simulink model "HW3-5"  (R2024b)
settings: Solver=FixedStepDiscrete  StartTime=0.0  StopTime=10  FixedStep=dt  RelTol=1e-3
PreLoadFcn:
  | run('params.m');
undefined symbols (not defined in the file or in its folder): DiscIntNeverNeededParam, dspblkCoreblockFVToolHelper, dt, gcbh, K1, K2, K3, r, R, tau1, tau2, tau3, th0, vx_d, vy_d, w_d, x0, y0
libraries: simulink x3, slpidlib x3
settings Model: Creator=obhav  LastModifiedBy=obhav
settings DataIOCC: ReturnWorkspaceOutputs=off

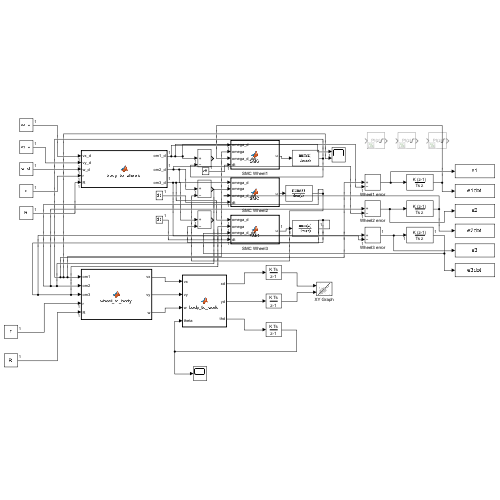
[thumbnail: Simulink's stored preview of the top-level diagram]
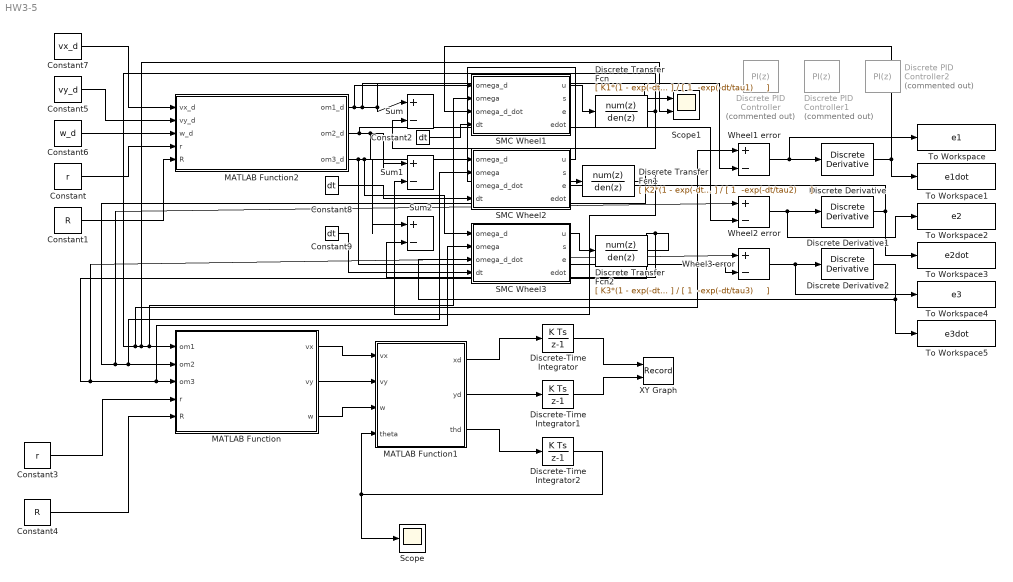
== system HW3-5 ==
  Constant : Constant  Value=r
  Constant1 : Constant  Value=R
  Constant2 : Constant  Value=dt
  Constant3 : Constant  Value=r
  Constant4 : Constant  Value=R
  Constant5 : Constant  Value=vy_d
  Constant6 : Constant  Value=w_d
  Constant7 : Constant  Value=vx_d
  Constant8 : Constant  Value=dt
  Constant9 : Constant  Value=dt
  Discrete Transfer Fcn : DiscreteTransferFcn  LoadFcn=dspblkCoreblockFVToolHelper(gcbh,'load');  Numerator=[ K1*(1 - exp(-dt/tau1)) ]  Denominator="[ 1  -exp(-dt/tau1)     ]"
      settings: CopyFcn=dspblkCoreblockFVToolHelper(gcbh,'copy');  DeleteFcn=dspblkCoreblockFVToolHelper(gcbh,'close');  ModelCloseFcn=dspblkCoreblockFVToolHelper(gcbh,'close');  PreSaveFcn=dspblkCoreblockFVToolHelper(gcbh,'presave');  PostSaveFcn=dspblkCoreblockFVToolHelper(gcbh,'postsave');  CloseFcn=dspblkCoreblockFVToolHelper(gcbh,'close');
  Discrete Transfer Fcn1 : DiscreteTransferFcn  LoadFcn=dspblkCoreblockFVToolHelper(gcbh,'load');  Numerator=[ K2*(1 - exp(-dt/tau2)) ]  Denominator="[ 1  -exp(-dt/tau2)     ]"
      settings: CopyFcn=dspblkCoreblockFVToolHelper(gcbh,'copy');  DeleteFcn=dspblkCoreblockFVToolHelper(gcbh,'close');  ModelCloseFcn=dspblkCoreblockFVToolHelper(gcbh,'close');  PreSaveFcn=dspblkCoreblockFVToolHelper(gcbh,'presave');  PostSaveFcn=dspblkCoreblockFVToolHelper(gcbh,'postsave');  CloseFcn=dspblkCoreblockFVToolHelper(gcbh,'close');
  Discrete Transfer Fcn2 : DiscreteTransferFcn  LoadFcn=dspblkCoreblockFVToolHelper(gcbh,'load');  Numerator=[ K3*(1 - exp(-dt/tau3)) ]  Denominator="[ 1  -exp(-dt/tau3)     ]"
      settings: CopyFcn=dspblkCoreblockFVToolHelper(gcbh,'copy');  DeleteFcn=dspblkCoreblockFVToolHelper(gcbh,'close');  ModelCloseFcn=dspblkCoreblockFVToolHelper(gcbh,'close');  PreSaveFcn=dspblkCoreblockFVToolHelper(gcbh,'presave');  PostSaveFcn=dspblkCoreblockFVToolHelper(gcbh,'postsave');  CloseFcn=dspblkCoreblockFVToolHelper(gcbh,'close');
  Discrete Derivative : simulink/Discrete/Discrete Derivative  gainval=1.0  ICPrevScaledInput=0.0  OutMin=[]  OutMax=[]  OutDataType=fixdt(1, 16)  OutScaling=2^-10  DoSatur=off
  Discrete Derivative1 : simulink/Discrete/Discrete Derivative  gainval=1.0  ICPrevScaledInput=0.0  OutMin=[]  OutMax=[]  OutDataType=fixdt(1, 16)  OutScaling=2^-10  DoSatur=off
  Discrete Derivative2 : simulink/Discrete/Discrete Derivative  gainval=1.0  ICPrevScaledInput=0.0  OutMin=[]  OutMax=[]  OutDataType=fixdt(1, 16)  OutScaling=2^-10  DoSatur=off
  Discrete PID Controller : slpidlib/PID Controller  Commented=on  Controller=PI  Form=Parallel  TimeDomain=Discrete-time  UseExternalTs=off  SampleTime=dt  IntegratorMethod=Forward Euler  FilterMethod=Forward Euler  ControllerParametersSource=internal  P=5  I=50  UseKiTs=off  D=0  UseExternalDerivativeSource=off  N=100  UseFilter=on  TunerSelectOption=Transfer Function Based (PID Tuner App)  InitialConditionSource=internal  InitialConditionForIntegrator=0  InitialConditionForFilter=0  DifferentiatorICPrevScaledInput=0  ExternalReset=none  TrackingMode=off  Kt=1  LimitOutput=on  SatLimitsSource=internal  UpperSaturationLimit=10  LowerSaturationLimit=-10  LinearizeAsGain=off  AntiWindupMode=clamping  Kb=1  LimitIntegrator=off  UpperIntegratorSaturationLimit=inf  LowerIntegratorSaturationLimit=-inf  POutMin=[]  POutMax=[]  IOutMin=[]  IOutMax=[]  DOutMin=[]  DOutMax=[]  NOutMin=[]  NOutMax=[]  SumOutMin=[]  SumOutMax=[]  SaturationOutMin=[]  SaturationOutMax=[]  PParamMin=[]  PParamMax=[]  IParamMin=[]  IParamMax=[]  DParamMin=[]  DParamMax=[]  NParamMin=[]  NParamMax=[]  KbParamMin=[]  KbParamMax=[]  KtParamMin=[]  KtParamMax=[]  KbOutMin=[]  KbOutMax=[]  KtOutMin=[]  KtOutMax=[]  IntegratorOutMin=[]  IntegratorOutMax=[]  FilterOutMin=[]  FilterOutMax=[]  SumI1OutMin=[]  SumI1OutMax=[]  SumI2OutMin=[]  SumI2OutMax=[]  SumI3OutMin=[]  SumI3OutMax=[]  SumI4OutMin=[]  SumI4OutMax=[]  SumDOutMin=[]  SumDOutMax=[]  DifferentiatorOutMin=[]  DifferentiatorOutMax=[]  FilterDiffOutCoefMin=[]  FilterDiffOutCoefMax=[]  ReciprocalOutMin=[]  ReciprocalOutMax=[]  SumDenOutMin=[]  SumDenOutMax=[]  SumNumOutMin=[]  SumNumOutMax=[]  DivideOutMin=[]  DivideOutMax=[]  UdiffTsProdOutMin=[]  UdiffTsProdOutMax=[]  NTsProdOutMin=[]  NTsProdOutMax=[]  UintegralTsProdOutMin=[]  UintegralTsProdOutMax=[]  UngainTsProdOutMin=[]  UngainTsProdOutMax=[]  ClampingZeroOutDataTypeStr=Inherit: Inherit via back propagation  ClampingZeroOutMin=[]  ClampingZeroOutMax=[]  FilterDenConstantOutDataTypeStr=Inherit: Inherit via back propagation  FilterDenConstantOutMin=[]  FilterDenConstantOutMax=[]  PCopyOutDataTypeStr=Inherit: Inherit via back propagation  PCopyOutMin=[]  PCopyOutMax=[]  NCopyOutDataTypeStr=Inherit: Inherit via back propagation  NCopyOutMin=[]  NCopyOutMax=[]  IntegratorContinuousStateAttributes=''  IntegratorStateMustResolveToSignalObject=off  IntegratorRTWStateStorageClass=Auto  FilterContinuousStateAttributes=''  FilterStateMustResolveToSignalObject=off  FilterRTWStateStorageClass=Auto  ParallelPVariant=InternalParameters  IdealPVariant=Disabled  IVariant=InternalParameters  DVariant=Disabled  IntegratorVariant=Discrete  SatVariant=Enabled  AWVariant=DiscClampingParallel  PCopyVariant=Disabled  TRVariant=Disabled  FdbkBlocksVariant=Forward  IdealPFdbkVariant=Disabled  SatFdbkVariant=Disabled  DerivativeFilterVariant=Disabled  NVariant=Disabled  NCopyVariant=Disabled_SignalSpec  FilterICVariant=Disabled  IntegratorICVariant=InternalICs  ExternalResetVariant=Disabled  TRSumVariant=Passthrough  SumFdbkVariant=Disabled  SumVariant=Sum_PI  TsampFilterVariant=InternalTs  TsampNgainVariant=Passthrough  TsampIntegralVariant=Disabled_SignalSpec  ExternalSaturationOutDataTypeStr=Inherit: Same as second input  DerivativeSourceVariant=Disabled  PreIntVariant=InternalPreInt
      settings: LibrarySourceBlock=simulink/Discrete/Discrete PID Controller
  Discrete PID Controller1 : slpidlib/PID Controller  Commented=on  Controller=PI  Form=Parallel  TimeDomain=Discrete-time  UseExternalTs=off  SampleTime=dt  IntegratorMethod=Forward Euler  FilterMethod=Forward Euler  ControllerParametersSource=internal  P=5  I=50  UseKiTs=off  D=0  UseExternalDerivativeSource=off  N=100  UseFilter=on  TunerSelectOption=Transfer Function Based (PID Tuner App)  InitialConditionSource=internal  InitialConditionForIntegrator=0  InitialConditionForFilter=0  DifferentiatorICPrevScaledInput=0  ExternalReset=none  TrackingMode=off  Kt=1  LimitOutput=on  SatLimitsSource=internal  UpperSaturationLimit=10  LowerSaturationLimit=-10  LinearizeAsGain=off  AntiWindupMode=clamping  Kb=1  LimitIntegrator=off  UpperIntegratorSaturationLimit=inf  LowerIntegratorSaturationLimit=-inf  POutMin=[]  POutMax=[]  IOutMin=[]  IOutMax=[]  DOutMin=[]  DOutMax=[]  NOutMin=[]  NOutMax=[]  SumOutMin=[]  SumOutMax=[]  SaturationOutMin=[]  SaturationOutMax=[]  PParamMin=[]  PParamMax=[]  IParamMin=[]  IParamMax=[]  DParamMin=[]  DParamMax=[]  NParamMin=[]  NParamMax=[]  KbParamMin=[]  KbParamMax=[]  KtParamMin=[]  KtParamMax=[]  KbOutMin=[]  KbOutMax=[]  KtOutMin=[]  KtOutMax=[]  IntegratorOutMin=[]  IntegratorOutMax=[]  FilterOutMin=[]  FilterOutMax=[]  SumI1OutMin=[]  SumI1OutMax=[]  SumI2OutMin=[]  SumI2OutMax=[]  SumI3OutMin=[]  SumI3OutMax=[]  SumI4OutMin=[]  SumI4OutMax=[]  SumDOutMin=[]  SumDOutMax=[]  DifferentiatorOutMin=[]  DifferentiatorOutMax=[]  FilterDiffOutCoefMin=[]  FilterDiffOutCoefMax=[]  ReciprocalOutMin=[]  ReciprocalOutMax=[]  SumDenOutMin=[]  SumDenOutMax=[]  SumNumOutMin=[]  SumNumOutMax=[]  DivideOutMin=[]  DivideOutMax=[]  UdiffTsProdOutMin=[]  UdiffTsProdOutMax=[]  NTsProdOutMin=[]  NTsProdOutMax=[]  UintegralTsProdOutMin=[]  UintegralTsProdOutMax=[]  UngainTsProdOutMin=[]  UngainTsProdOutMax=[]  ClampingZeroOutDataTypeStr=Inherit: Inherit via back propagation  ClampingZeroOutMin=[]  ClampingZeroOutMax=[]  FilterDenConstantOutDataTypeStr=Inherit: Inherit via back propagation  FilterDenConstantOutMin=[]  FilterDenConstantOutMax=[]  PCopyOutDataTypeStr=Inherit: Inherit via back propagation  PCopyOutMin=[]  PCopyOutMax=[]  NCopyOutDataTypeStr=Inherit: Inherit via back propagation  NCopyOutMin=[]  NCopyOutMax=[]  IntegratorContinuousStateAttributes=''  IntegratorStateMustResolveToSignalObject=off  IntegratorRTWStateStorageClass=Auto  FilterContinuousStateAttributes=''  FilterStateMustResolveToSignalObject=off  FilterRTWStateStorageClass=Auto  ParallelPVariant=InternalParameters  IdealPVariant=Disabled  IVariant=InternalParameters  DVariant=Disabled  IntegratorVariant=Discrete  SatVariant=Enabled  AWVariant=DiscClampingParallel  PCopyVariant=Disabled  TRVariant=Disabled  FdbkBlocksVariant=Forward  IdealPFdbkVariant=Disabled  SatFdbkVariant=Disabled  DerivativeFilterVariant=Disabled  NVariant=Disabled  NCopyVariant=Disabled_SignalSpec  FilterICVariant=Disabled  IntegratorICVariant=InternalICs  ExternalResetVariant=Disabled  TRSumVariant=Passthrough  SumFdbkVariant=Disabled  SumVariant=Sum_PI  TsampFilterVariant=InternalTs  TsampNgainVariant=Passthrough  TsampIntegralVariant=Disabled_SignalSpec  ExternalSaturationOutDataTypeStr=Inherit: Same as second input  DerivativeSourceVariant=Disabled  PreIntVariant=InternalPreInt
      settings: LibrarySourceBlock=simulink/Discrete/Discrete PID Controller
  Discrete PID Controller2 : slpidlib/PID Controller  Commented=on  Controller=PI  Form=Parallel  TimeDomain=Discrete-time  UseExternalTs=off  SampleTime=dt  IntegratorMethod=Forward Euler  FilterMethod=Forward Euler  ControllerParametersSource=internal  P=5  I=50  UseKiTs=off  D=0  UseExternalDerivativeSource=off  N=100  UseFilter=on  TunerSelectOption=Transfer Function Based (PID Tuner App)  InitialConditionSource=internal  InitialConditionForIntegrator=0  InitialConditionForFilter=0  DifferentiatorICPrevScaledInput=0  ExternalReset=none  TrackingMode=off  Kt=1  LimitOutput=on  SatLimitsSource=internal  UpperSaturationLimit=10  LowerSaturationLimit=-10  LinearizeAsGain=off  AntiWindupMode=clamping  Kb=1  LimitIntegrator=off  UpperIntegratorSaturationLimit=inf  LowerIntegratorSaturationLimit=-inf  POutMin=[]  POutMax=[]  IOutMin=[]  IOutMax=[]  DOutMin=[]  DOutMax=[]  NOutMin=[]  NOutMax=[]  SumOutMin=[]  SumOutMax=[]  SaturationOutMin=[]  SaturationOutMax=[]  PParamMin=[]  PParamMax=[]  IParamMin=[]  IParamMax=[]  DParamMin=[]  DParamMax=[]  NParamMin=[]  NParamMax=[]  KbParamMin=[]  KbParamMax=[]  KtParamMin=[]  KtParamMax=[]  KbOutMin=[]  KbOutMax=[]  KtOutMin=[]  KtOutMax=[]  IntegratorOutMin=[]  IntegratorOutMax=[]  FilterOutMin=[]  FilterOutMax=[]  SumI1OutMin=[]  SumI1OutMax=[]  SumI2OutMin=[]  SumI2OutMax=[]  SumI3OutMin=[]  SumI3OutMax=[]  SumI4OutMin=[]  SumI4OutMax=[]  SumDOutMin=[]  SumDOutMax=[]  DifferentiatorOutMin=[]  DifferentiatorOutMax=[]  FilterDiffOutCoefMin=[]  FilterDiffOutCoefMax=[]  ReciprocalOutMin=[]  ReciprocalOutMax=[]  SumDenOutMin=[]  SumDenOutMax=[]  SumNumOutMin=[]  SumNumOutMax=[]  DivideOutMin=[]  DivideOutMax=[]  UdiffTsProdOutMin=[]  UdiffTsProdOutMax=[]  NTsProdOutMin=[]  NTsProdOutMax=[]  UintegralTsProdOutMin=[]  UintegralTsProdOutMax=[]  UngainTsProdOutMin=[]  UngainTsProdOutMax=[]  ClampingZeroOutDataTypeStr=Inherit: Inherit via back propagation  ClampingZeroOutMin=[]  ClampingZeroOutMax=[]  FilterDenConstantOutDataTypeStr=Inherit: Inherit via back propagation  FilterDenConstantOutMin=[]  FilterDenConstantOutMax=[]  PCopyOutDataTypeStr=Inherit: Inherit via back propagation  PCopyOutMin=[]  PCopyOutMax=[]  NCopyOutDataTypeStr=Inherit: Inherit via back propagation  NCopyOutMin=[]  NCopyOutMax=[]  IntegratorContinuousStateAttributes=''  IntegratorStateMustResolveToSignalObject=off  IntegratorRTWStateStorageClass=Auto  FilterContinuousStateAttributes=''  FilterStateMustResolveToSignalObject=off  FilterRTWStateStorageClass=Auto  ParallelPVariant=InternalParameters  IdealPVariant=Disabled  IVariant=InternalParameters  DVariant=Disabled  IntegratorVariant=Discrete  SatVariant=Enabled  AWVariant=DiscClampingParallel  PCopyVariant=Disabled  TRVariant=Disabled  FdbkBlocksVariant=Forward  IdealPFdbkVariant=Disabled  SatFdbkVariant=Disabled  DerivativeFilterVariant=Disabled  NVariant=Disabled  NCopyVariant=Disabled_SignalSpec  FilterICVariant=Disabled  IntegratorICVariant=InternalICs  ExternalResetVariant=Disabled  TRSumVariant=Passthrough  SumFdbkVariant=Disabled  SumVariant=Sum_PI  TsampFilterVariant=InternalTs  TsampNgainVariant=Passthrough  TsampIntegralVariant=Disabled_SignalSpec  ExternalSaturationOutDataTypeStr=Inherit: Same as second input  DerivativeSourceVariant=Disabled  PreIntVariant=InternalPreInt
      settings: LibrarySourceBlock=simulink/Discrete/Discrete PID Controller
  Discrete-Time Integrator : DiscreteIntegrator  InitialCondition=x0  SampleTime=dt  ICPrevOutput=DiscIntNeverNeededParam  ICPrevScaledInput=DiscIntNeverNeededParam
  Discrete-Time Integrator1 : DiscreteIntegrator  InitialCondition=y0  SampleTime=dt  ICPrevOutput=DiscIntNeverNeededParam  ICPrevScaledInput=DiscIntNeverNeededParam
  Discrete-Time Integrator2 : DiscreteIntegrator  InitialCondition=th0  SampleTime=dt  ICPrevOutput=DiscIntNeverNeededParam  ICPrevScaledInput=DiscIntNeverNeededParam
  MATLAB Function : MATLAB Function  TreatAsAtomicUnit=on
  MATLAB Function1 : MATLAB Function  TreatAsAtomicUnit=on
  MATLAB Function2 : MATLAB Function  TreatAsAtomicUnit=on
  SMC Wheel1 : MATLAB Function  TreatAsAtomicUnit=on
  SMC Wheel2 : MATLAB Function  TreatAsAtomicUnit=on
  SMC Wheel3 : MATLAB Function  TreatAsAtomicUnit=on
  Scope : Scope
  Scope1 : Scope  NumInputPorts=2
  Sum : Sum  Inputs=|+-
  Sum1 : Sum  Inputs=|+-
  Sum2 : Sum  Inputs=|+-
  To Workspace : ToWorkspace  VariableName=e1  SampleTime=-1
  To Workspace1 : ToWorkspace  VariableName=e1dot  SampleTime=-1
  To Workspace2 : ToWorkspace  VariableName=e2  SampleTime=-1
  To Workspace3 : ToWorkspace  VariableName=e2dot  SampleTime=-1
  To Workspace4 : ToWorkspace  VariableName=e3  SampleTime=-1
  To Workspace5 : ToWorkspace  VariableName=e3dot  SampleTime=-1
  Wheel1 error : Sum  Inputs=|+-
  Wheel2 error : Sum  Inputs=|+-
  Wheel3 error : Sum  Inputs=|+-
  XY Graph : Record  FileSettingsInternal="{\"entries\":[{\"content\":{\"excelSettings\":{\"content\":{},\"type\":\"Streamout.ExcelSettings\"}},\"type\":\"Streamout.FileSettingStorage\",\"uuid\":\"\"}],\"packageUris\":[\"http:\\/\\/schema.mathworks.com\\/mf0\\/streamout_blocks\\/R2020a\"],\"version\":\"1.0\"}"  Layout=[1 1]  SignalsInternal="{\"entries\":[{\"content\":{\"signals\":[{\"content\":{\"blockPath\":[],\"dimensions\":[1],\"domain\":\"\",\"lineColor\":\"#a2142f\",\"plots\":[ 1 ],\"port\":1,\"sid\":[\"\"],\"signalID\":1,\"signalName\":\"Discrete-Time\\nIntegrator\"},\"type\":\"RecordBlkView.Signal\",\"uuid\":\"\"},{\"content\":{\"blockPath\":[],\"dimensions\":[1],\"domain\":\"\",\"lineColor\":\"#139fff\",\"plots\":[ 1 ],\"port\":2,\"sid\":[\"\"],\"signalID\":2,\"signalName\":\"Discrete-Time\\nIntegrator1\"},\"type\":\"RecordBlkView.Signal\",\"uuid\":\"\"}]},\"type\":\"RecordBlkView.InputSignals\",\"uuid\":\"\"}],\"packageUris\":[\"http:\\/\\/schema.mathworks.com\\/mf0\\/streamout_blocks\\/R2020a\"],\"version\":\"1.0\"}"  VisualizationBindings="{\"xyplotplugin\":{\"info\":[{\"series\":[{\"bindingParametersList\":[{\"parameter\":\"X-Axis\",\"signalID\":1,\"signalName\":\"Discrete-Time\\nIntegrator\"},{\"parameter\":\"Y-Axis\",\"signalID\":2,\"signalName\":\"Discrete-Time\\nIntegrator1\"}],\"seriesID\":0}],\"subplotID\":1}]}}"  CompatibilityTag=XY
  wires:
  Discrete-Time Integrator/1 -> XY Graph/1
  Discrete-Time Integrator1/1 -> XY Graph/2
  MATLAB Function1/1(xd) -> Discrete-Time Integrator/1
  MATLAB Function1/2(yd) -> Discrete-Time Integrator1/1
  MATLAB Function1/3(thd) -> Discrete-Time Integrator2/1
  Discrete-Time Integrator2/1 -> MATLAB Function1/4(theta), Scope/1
  MATLAB Function/3(w) -> MATLAB Function1/3(w)
  MATLAB Function/2(vy) -> MATLAB Function1/2(vy)
  MATLAB Function/1(vx) -> MATLAB Function1/1(vx)
  Constant3/1 -> MATLAB Function/4(r)
  Constant4/1 -> MATLAB Function/5(R)
  Constant7/1 -> MATLAB Function2/1(vx_d)
  Constant5/1 -> MATLAB Function2/2(vy_d)
  Constant6/1 -> MATLAB Function2/3(w_d)
  Constant/1 -> MATLAB Function2/4(r)
  Constant1/1 -> MATLAB Function2/5(R)
  MATLAB Function2/1(om1_d) -> SMC Wheel1/1(omega_d), Wheel1 error/2, Scope1/1, Sum/1
  MATLAB Function2/2(om2_d) -> Wheel2 error/2, SMC Wheel2/1(omega_d), Sum1/1
  MATLAB Function2/3(om3_d) -> Wheel3 error/2, SMC Wheel3/1(omega_d), Sum2/1
  Discrete Transfer Fcn/1 -> Wheel1 error/1, Scope1/2, SMC Wheel1/2(omega), MATLAB Function/1(om1), Sum/2
  Discrete Transfer Fcn1/1 -> SMC Wheel2/2(omega), MATLAB Function/2(om2), Wheel2 error/1, Sum1/2
  Discrete Transfer Fcn2/1 -> Wheel3 error/1, SMC Wheel3/2(omega), MATLAB Function/3(om3), Sum2/2
  Wheel1 error/1 -> To Workspace/1, Discrete Derivative/1
  Wheel2 error/1 -> To Workspace2/1, Discrete Derivative1/1
  Wheel3 error/1 -> To Workspace4/1, Discrete Derivative2/1
  Discrete Derivative/1 -> To Workspace1/1, SMC Wheel1/3(omega_d_dot)
  Discrete Derivative1/1 -> To Workspace3/1, SMC Wheel2/3(omega_d_dot)
  Discrete Derivative2/1 -> SMC Wheel3/3(omega_d_dot), To Workspace5/1
  SMC Wheel1/1(u) -> Discrete Transfer Fcn/1
  SMC Wheel2/1(u) -> Discrete Transfer Fcn1/1
  SMC Wheel3/1(u) -> Discrete Transfer Fcn2/1
  Constant2/1 -> SMC Wheel1/4(dt)
  Constant8/1 -> SMC Wheel2/4(dt)
  Constant9/1 -> SMC Wheel3/4(dt)

== matlab function HW3-5/MATLAB Function1 ==
  data: vx input; xd output; vy input; w input; theta input; yd output; thd output
function [xd, yd, thd] = body_to_world(vx, vy, w, theta)
xd  =  vx*cos(theta) - vy*sin(theta);
yd  =  vx*sin(theta) + vy*cos(theta);
thd =  w;
end

== matlab function HW3-5/MATLAB Function ==
  data: om1 input; vx output; om2 input; om3 input; r input; R input; vy output; w output
function [vx, vy, w] = wheel_to_body(om1, om2, om3, r, R)
vx = (r/sqrt(3))*(-om2 + om3);
vy = (r/3)*(2*om1 - om2 - om3);
w  = (r/(3*R))*(om1 + om2 + om3);
end

== matlab function HW3-5/MATLAB Function2 ==
  data: vx_d input; om1_d output; vy_d input; w_d input; r input; R input; om2_d output; om3_d output
function [om1_d, om2_d, om3_d] = body_to_wheels(vx_d, vy_d, w_d, r, R)
%#codegen
% A = [ -sinφ  cosφ  R ] rows with φ1=0, φ2=120°, φ3=240°
% Closed-form for 120° geometry:
om1_d = (vy_d + R*w_d) / r;
om2_d = ( -sqrt(3)/2*vx_d - 1/2*vy_d + R*w_d ) / r;
om3_d = (  sqrt(3)/2*vx_d - 1/2*vy_d + R*w_d ) / r;
end

== matlab function HW3-5/SMC Wheel1 ==
  data: omega_d input; u output; omega input; omega_d_dot input; dt input; s output; e output; edot output
function [u, s, e, edot] = SMC_Controller(omega_d, omega, omega_d_dot, dt)
%#codegen

% outputs to initialize
u    = 0.0;
s    = 0.0;
e    = 0.0;
edot = 0.0;

%  gains (tune) 
c   = 5.0;     % sliding surface gain
k   = 2.0;     % switching gain
phi = 0.05;    % smoothing for tanh to avoid chattering

% discrete derivative of omega (using dt) 
persistent omega_prev
if isempty(omega_prev)
    omega_prev = omega;
end

e    = omega_d - omega;
edot = omega_d_dot - (omega - omega_prev)/dt;

% sliding surface
s = c*e + edot;

% control (equivalent + switching; you may use c*e or c*edot depending on design)
u = c*e + k*tanh(s/phi);
% alternative:  u = -k*sign(s) + c*e;

omega_prev = omega;
end

== matlab function HW3-5/SMC Wheel2 ==
  data: omega_d input; u output; omega input; omega_d_dot input; dt input; s output; e output; edot output
function [u, s, e, edot] = SMC_Controller(omega_d, omega, omega_d_dot, dt)
%#codegen

% ---- outputs must be scalars (initialize) ----
u    = 0.0;
s    = 0.0;
e    = 0.0;
edot = 0.0;

% ---- gains (tune) ----
c   = 5.0;     % sliding surface gain
k   = 2.0;     % switching gain
phi = 0.05;    % smoothing for tanh to avoid chattering

% ---- discrete derivative of omega (using dt) ----
persistent omega_prev
if isempty(omega_prev)
    omega_prev = omega;
end

e    = omega_d - omega;
edot = omega_d_dot - (omega - omega_prev)/dt;

% sliding surface
s = c*e + edot;

% control (equivalent + switching; you may use c*e or c*edot depending on design)
u = c*e + k*tanh(s/phi);
% alternative:  u = -k*sign(s) + c*e;

omega_prev = omega;
end

== matlab function HW3-5/SMC Wheel3 ==
  data: omega_d input; u output; omega input; omega_d_dot input; dt input; s output; e output; edot output
function [u, s, e, edot] = SMC_Controller(omega_d, omega, omega_d_dot, dt)
%#codegen

% ---- outputs must be scalars (initialize) ----
u    = 0.0;
s    = 0.0;
e    = 0.0;
edot = 0.0;

% ---- gains (tune) ----
c   = 5.0;     % sliding surface gain
k   = 2.0;     % switching gain
phi = 0.05;    % smoothing for tanh to avoid chattering

% ---- discrete derivative of omega (using dt) ----
persistent omega_prev
if isempty(omega_prev)
    omega_prev = omega;
end

e    = omega_d - omega;
edot = omega_d_dot - (omega - omega_prev)/dt;

% sliding surface
s = c*e + edot;

% control (equivalent + switching; you may use c*e or c*edot depending on design)
u = c*e + k*tanh(s/phi);
% alternative:  u = -k*sign(s) + c*e;

omega_prev = omega;
end
